simulink model "Model2"  (R2020a)
settings: Solver=VariableStepAuto  StartTime=0.0  StopTime=10.0  RelTol=1e-3
undefined symbols (not defined in the file): b, K1, K2, M1, M2
settings Model: Creator=HP  LastModifiedBy=HP

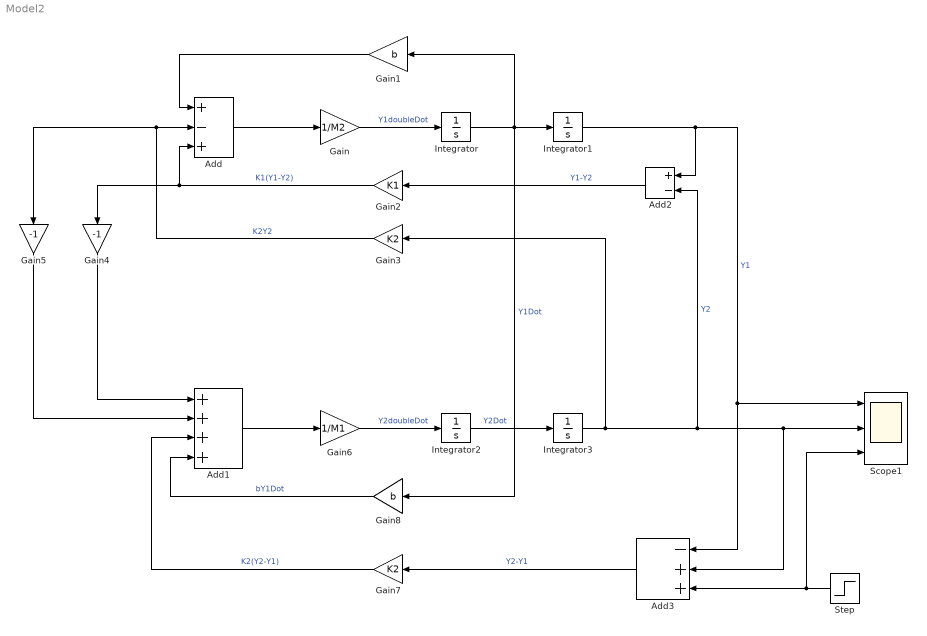
== system Model2 ==
  Add : Sum  Inputs=+-+
  Add1 : Sum  Inputs=++++
  Add2 : Sum  Inputs=+-
  Add3 : Sum  Inputs=-++
  Gain : Gain  Gain=1/M2
  Gain1 : Gain  Gain=b
  Gain2 : Gain  Gain=K1
  Gain3 : Gain  Gain=K2
  Gain4 : Gain  Gain=-1
  Gain5 : Gain  Gain=-1
  Gain6 : Gain  Gain=1/M1
  Gain7 : Gain  Gain=K2
  Gain8 : Gain  Gain=b
  Integrator{,1..3} (4 alike) : Integrator
  Scope1 : Scope  NumInputPorts=3
  Step : Step  SampleTime=0
  wires:
  Integrator1/1 -> Add2/1, Add3/1, Scope1/1  "Y1"
  Integrator/1 -> Integrator1/1, Gain8/1, Gain1/1  "Y1Dot"
  Gain/1 -> Integrator/1  "Y1doubleDot"
  Add/1 -> Gain/1
  Gain1/1 -> Add/1
  Add2/1 -> Gain2/1  "Y1-Y2"
  Gain2/1 -> Gain4/1, Add/3  "K1(Y1-Y2)"
  Gain3/1 -> Add/2, Gain5/1  "K2Y2"
  Integrator2/1 -> Integrator3/1  "Y2Dot"
  Gain6/1 -> Integrator2/1  "Y2doubleDot"
  Add1/1 -> Gain6/1
  Integrator3/1 -> Gain3/1, Add2/2, Scope1/2, Add3/2  "Y2"
  Step/1 -> Scope1/3, Add3/3
  Add3/1 -> Gain7/1  "Y2-Y1"
  Gain4/1 -> Add1/1
  Gain5/1 -> Add1/2
  Gain8/1 -> Add1/4  "bY1Dot"
  Gain7/1 -> Add1/3  "K2(Y2-Y1)"
